simulink model "BodyDynamics"  (R2022b)
settings: Solver=VariableStepAuto  StartTime=0.0  StopTime=60  RelTol=1e-3
values from neighbouring files (symbols this model uses):
  csi_0 = [x_0, z_0, theta_0, u_0, w_0, q_0]'    [Inizializzazione.m]
  dt = double(subs(dt,dt, 0.01))    [Inizializzazione.m]
  is_particle = true    [Inizializzazione.m]
  P_00 = diag([0.1,0.1,0.1,0.1,0.1,0.1])    [Inizializzazione.m]
  Q = diag([var_tau_u, var_tau_w, var_tau_q])    [Inizializzazione.m]
  q_0 = 0    [Inizializzazione.m]
  R = diag([var_y_alpha_m, var_z_m, var_theta_m])    [Inizializzazione.m]
  S = [m , I_y, Damping_matrix(1,1), Damping_matrix(2,2), Damping_matrix(3,3)]    [Inizializzazione.m]
  theta_0 = wrapTo2Pi(rand() * (pi/2) - pi)    [Inizializzazione.m]
  u_0 = 0    [Inizializzazione.m]
  w_0 = 0    [Inizializzazione.m]
  x_0 = rand() * x_boa_1*3/4    [Inizializzazione.m]
  z_0 = rand() * z_boa_2*3/4    [Inizializzazione.m]
  z_boa_2 = 150    [Inizializzazione.m]
libraries: simulink x6
settings Model: Creator=angel  LastModifiedBy=angel
settings DebuggingCC: UnderSpecifiedDimensionMsg=warning
settings ModelReferenceCC: EnableRefExpFcnMdlSchedulingChecks=on

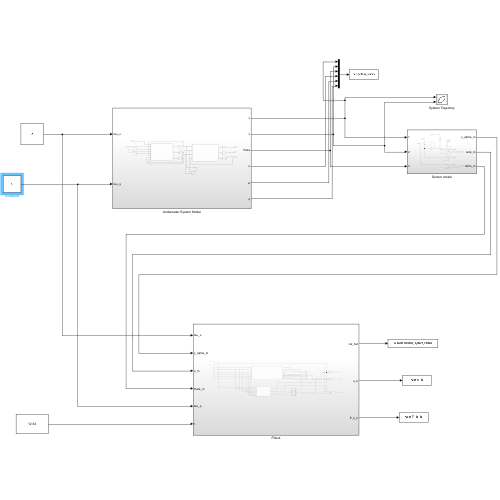
[thumbnail: Simulink's stored preview of the top-level diagram]
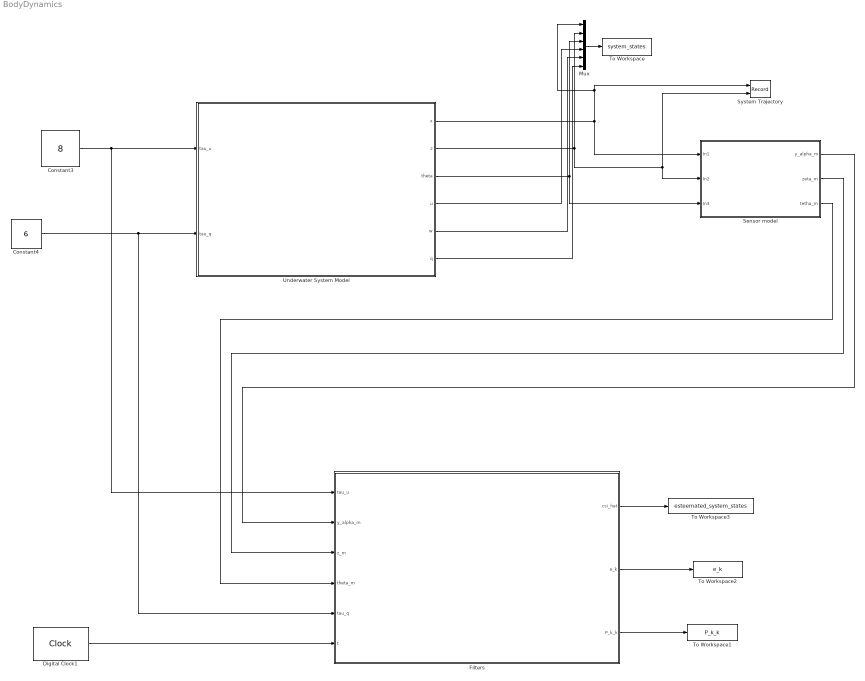
== system BodyDynamics ==
  Constant3 : Constant  Value=8
  Constant4 : Constant  Value=6
  Digital Clock1 : DigitalClock  SampleTime=0.1
  Filters : Subsystem
  Mux : Mux  Inputs=6
  Sensor model : Subsystem
  System Trajectory : Record  FileSettingsInternal="{\"entries\":[{\"content\":{\"excelSettings\":{\"content\":{},\"type\":\"Streamout.ExcelSettings\"}},\"type\":\"Streamout.FileSettingStorage\",\"uuid\":\"5a9cd2f8-3f1b-4377-9d18-0cf4235dc122\"}],\"packageUris\":[\"http://schema.mathworks.com/mf0/streamout_blocks/R2020a\"],\"version\":\"1.0\"}"  Layout=[1 1]  SignalsInternal="{\"entries\":[{\"content\":{\"signals\":[{\"content\":{\"blockPath\":[\"BodyDynamics/System Trajectory\"],\"channel\":[],\"dimensions\":[1],\"domain\":\"BodyDynamics/System Trajectory\",\"lineColor\":\"#ff6929\",\"plots\":[],\"port\":1,\"sid\":[\"\"],\"signalID\":475,\"signalName\":\"Underwater System Model:1\"},\"type\":\"RecordBlkView.Signal\",\"uuid\":\"2e985c3f-a8fe-4c9c-bedf-405b71b3ce1e\"},{\"content\":{\"blockPath\":[\"BodyDynamics/System Trajectory\"],\"channel\":[],\"dimensions\":[1],\"domain\":\"BodyDynamics/System Trajectory\",\"lineColor\":\"#b746ff\",\"plots\":[],\"port\":2,\"sid\":[\"\"],\"signalID\":479,\"signalName\":\"Underwater System Model:2\"},\"type\":\"RecordBlkView.Signal\",\"uuid\":\"8a6af6fa-3ed6-44e8-a576-d0f0524b2a32\"}]},\"type\":\"RecordBlkView.InputSignals\",\"uuid\":\"c673d974-d470-40e6-a6d2-e1dc34d32e7d\"}],\"packageUris\":[\"http://schema.mathworks.com/mf0/streamout_blocks/R2020a\"],\"version\":\"1.0\"}"  VisualizationBindings="{\"xyplotplugin\":{\"info\":[{\"series\":[],\"subplotID\":1}]}}"  CompatibilityTag=XY
  To Workspace : ToWorkspace  VariableName=system_states  SampleTime=dt
  To Workspace1 : ToWorkspace  VariableName=P_k_k  SampleTime=dt
  To Workspace2 : ToWorkspace  VariableName=e_k  SampleTime=dt
  To Workspace3 : ToWorkspace  VariableName=esteemated_system_states  SampleTime=dt
  Underwater System Model : Subsystem
  wires:
  Underwater System Model/1(x) -> System Trajectory/1, Mux/1, Sensor model/1(In1)
  Underwater System Model/2(z) -> System Trajectory/2, Sensor model/2(In2), Mux/2
  Underwater System Model/3(theta) -> Sensor model/3(In3), Mux/3
  Underwater System Model/4(u) -> Mux/4
  Underwater System Model/5(w) -> Mux/5
  Underwater System Model/6(q) -> Mux/6
  Mux/1 -> To Workspace/1
  Constant3/1 -> Filters/1(tau_u), Underwater System Model/1(tau_u)
  Constant4/1 -> Filters/5(tau_q), Underwater System Model/2(tau_q)
  Sensor model/1(y_alpha_m) -> Filters/2(y_alpha_m)
  Sensor model/2(zeta_m) -> Filters/3(z_m)
  Sensor model/3(tetha_m) -> Filters/4(theta_m)
  Digital Clock1/1 -> Filters/6(t)
  Filters/1(csi_hat) -> To Workspace3/1
  Filters/2(e_k) -> To Workspace2/1
  Filters/3(P_k_k) -> To Workspace1/1

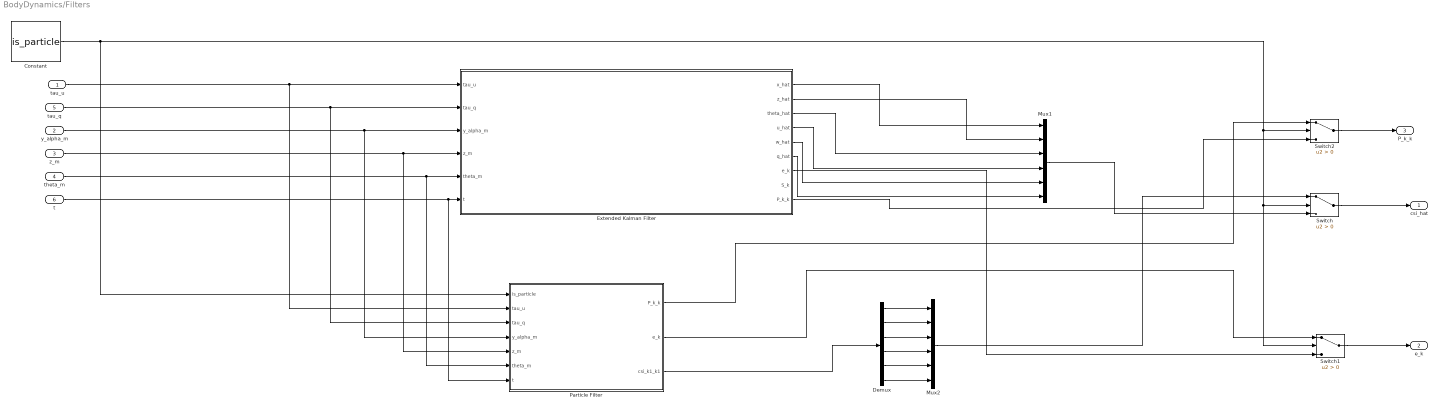
== system BodyDynamics/Filters ==
  tau_u : Inport
  y_alpha_m : Inport  Port=2
  z_m : Inport  Port=3
  theta_m : Inport  Port=4
  tau_q : Inport  Port=5
  t : Inport  Port=6
  Constant : Constant  Value=is_particle
  Demux : Demux  Outputs=6
  Extended Kalman Filter : Subsystem
  Mux1 : Mux  Inputs=6
  Mux2 : Mux  Inputs=6
  Particle Filter : Subsystem
  Switch : Switch  Criteria=u2 > Threshold  SaturateOnIntegerOverflow=off  InputSameDT=off
  Switch1 : Switch  Criteria=u2 > Threshold  SaturateOnIntegerOverflow=off  InputSameDT=off
  Switch2 : Switch  Criteria=u2 > Threshold  SaturateOnIntegerOverflow=off  InputSameDT=off
  csi_hat : Outport
  e_k : Outport  Port=2
  P_k_k : Outport  Port=3
  wires:
  Extended Kalman Filter/4(u_hat) -> Mux1/4
  Extended Kalman Filter/1(x_hat) -> Mux1/1
  Extended Kalman Filter/5(w_hat) -> Mux1/5
  Extended Kalman Filter/2(z_hat) -> Mux1/2
  Demux/4 -> Mux2/4
  Demux/2 -> Mux2/2
  Extended Kalman Filter/6(q_hat) -> Mux1/6
  Demux/6 -> Mux2/6
  Demux/3 -> Mux2/3
  Demux/1 -> Mux2/1
  Extended Kalman Filter/3(theta_hat) -> Mux1/3
  Demux/5 -> Mux2/5
  Mux2/1 -> Switch/1
  Mux1/1 -> Switch/3
  Switch/1 -> csi_hat/1
  Extended Kalman Filter/7(e_k) -> Switch1/3
  Switch1/1 -> e_k/1
  Constant/1 -> Particle Filter/1(is_particle), Switch1/2, Switch/2, Switch2/2
  tau_u/1 -> Particle Filter/2(tau_u), Extended Kalman Filter/1(tau_u)
  tau_q/1 -> Particle Filter/3(tau_q), Extended Kalman Filter/2(tau_q)
  y_alpha_m/1 -> Particle Filter/4(y_alpha_m), Extended Kalman Filter/3(y_alpha_m)
  z_m/1 -> Particle Filter/5(z_m), Extended Kalman Filter/4(z_m)
  theta_m/1 -> Particle Filter/6(theta_m), Extended Kalman Filter/5(theta_m)
  t/1 -> Particle Filter/7(t), Extended Kalman Filter/6(t)
  Extended Kalman Filter/9(P_k_k) -> Switch2/3
  Switch2/1 -> P_k_k/1
  Particle Filter/1(P_k_k) -> Switch2/1
  Particle Filter/2(e_k) -> Switch1/1
  Particle Filter/3(csi_k1_k1) -> Demux/1

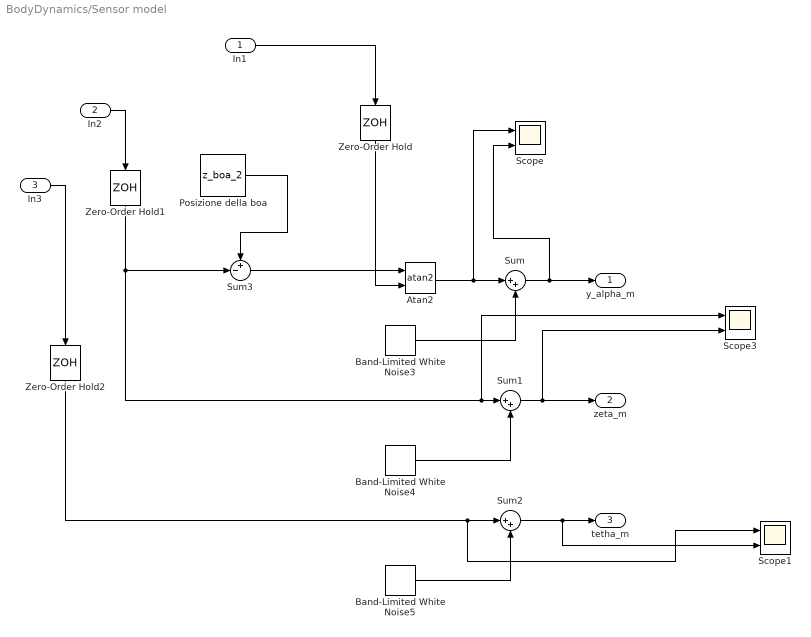
== system BodyDynamics/Sensor model ==
  In1 : Inport
  In2 : Inport  Port=2
  In3 : Inport  Port=3
  Atan2 : Trigonometry  Operator=atan2
  Band-Limited White Noise3 : simulink/Sources/Band-Limited White Noise  Cov=var_y_alpha_m  Ts=dt  seed=[23341]
  Band-Limited White Noise4 : simulink/Sources/Band-Limited White Noise  Cov=var_z_m  Ts=dt  seed=[23341]
  Band-Limited White Noise5 : simulink/Sources/Band-Limited White Noise  Cov=var_theta_m  Ts=dt  seed=[23341]
  Posizione della boa : Constant  Value=z_boa_2
  Scope : Scope  NumInputPorts=2
  Scope1 : Scope  NumInputPorts=2
  Scope3 : Scope  NumInputPorts=2
  Sum : Sum  Inputs=|++
  Sum1 : Sum  Inputs=|++
  Sum2 : Sum  Inputs=|++
  Sum3 : Sum  Inputs=+-|
  Zero-Order Hold : ZeroOrderHold  SampleTime=dt
  Zero-Order Hold1 : ZeroOrderHold  SampleTime=dt
  Zero-Order Hold2 : ZeroOrderHold  SampleTime=dt
  y_alpha_m : Outport
  zeta_m : Outport  Port=2
  tetha_m : Outport  Port=3
  wires:
  In3/1 -> Zero-Order Hold2/1
  In1/1 -> Zero-Order Hold/1
  Sum2/1 -> Scope1/2, tetha_m/1
  Sum1/1 -> Scope3/2, zeta_m/1
  In2/1 -> Zero-Order Hold1/1
  Band-Limited White Noise3/1 -> Sum/2
  Band-Limited White Noise4/1 -> Sum1/2
  Band-Limited White Noise5/1 -> Sum2/2
  Zero-Order Hold/1 -> Atan2/2
  Zero-Order Hold1/1 -> Sum3/2, Scope3/1, Sum1/1
  Zero-Order Hold2/1 -> Scope1/1, Sum2/1
  Posizione della boa/1 -> Sum3/1
  Sum3/1 -> Atan2/1
  Atan2/1 -> Scope/1, Sum/1
  Sum/1 -> y_alpha_m/1, Scope/2

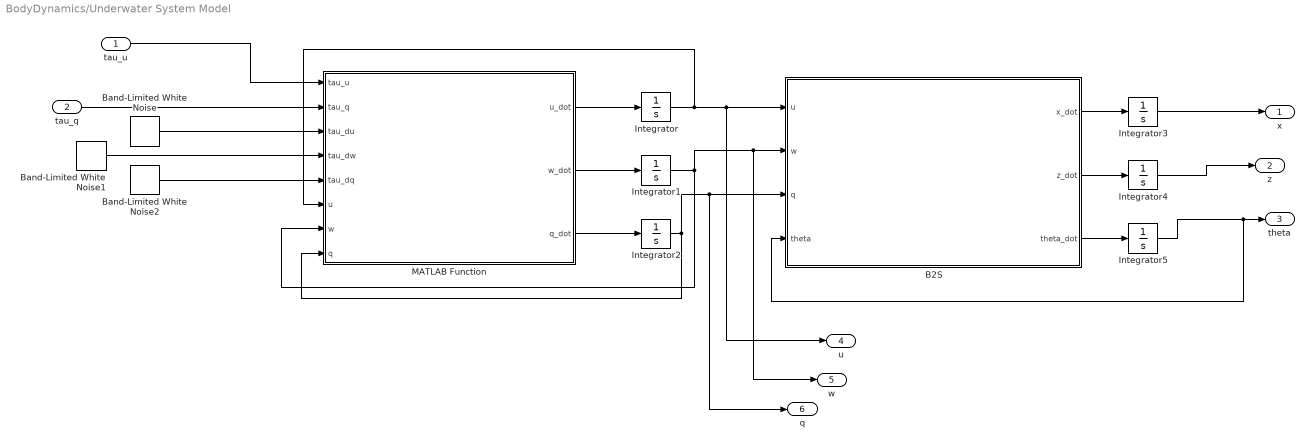
== system BodyDynamics/Underwater System Model ==
  tau_u : Inport
  tau_q : Inport  Port=2
  B2S : MATLAB Function  TreatAsAtomicUnit=on
  Band-Limited White Noise : simulink/Sources/Band-Limited White Noise  Cov=var_tau_u  Ts=dt  seed=[23341]
  Band-Limited White Noise1 : simulink/Sources/Band-Limited White Noise  Cov=var_tau_w  Ts=dt  seed=[23341]
  Band-Limited White Noise2 : simulink/Sources/Band-Limited White Noise  Cov=var_tau_q  Ts=dt  seed=[23341]
  Integrator : Integrator  InitialCondition=u_0
  Integrator1 : Integrator  InitialCondition=w_0
  Integrator2 : Integrator  InitialCondition=q_0
  Integrator3 : Integrator  InitialCondition=x_0
  Integrator4 : Integrator  InitialCondition=z_0
  Integrator5 : Integrator  InitialCondition=theta_0  WrappedStateUpperValue=2*pi  WrappedStateLowerValue=0
  MATLAB Function : MATLAB Function  TreatAsAtomicUnit=on  mask{S=S}
      mask prompts: S "Costanti del sistema"
  x : Outport
  z : Outport  Port=2
  theta : Outport  Port=3
  u : Outport  Port=4
  w : Outport  Port=5
  q : Outport  Port=6
  wires:
  B2S/2(z_dot) -> Integrator4/1
  Integrator1/1 -> MATLAB Function/7(w), w/1, B2S/2(w)
  Band-Limited White Noise2/1 -> MATLAB Function/5(tau_dq)
  B2S/3(theta_dot) -> Integrator5/1
  MATLAB Function/2(w_dot) -> Integrator1/1
  Integrator/1 -> MATLAB Function/6(u), B2S/1(u), u/1
  B2S/1(x_dot) -> Integrator3/1
  MATLAB Function/3(q_dot) -> Integrator2/1
  MATLAB Function/1(u_dot) -> Integrator/1
  Band-Limited White Noise1/1 -> MATLAB Function/4(tau_dw)
  tau_u/1 -> MATLAB Function/1(tau_u)
  Integrator2/1 -> MATLAB Function/8(q), q/1, B2S/3(q)
  Band-Limited White Noise/1 -> MATLAB Function/3(tau_du)
  Integrator5/1 -> B2S/4(theta), theta/1
  Integrator3/1 -> x/1
  Integrator4/1 -> z/1
  tau_q/1 -> MATLAB Function/2(tau_q)

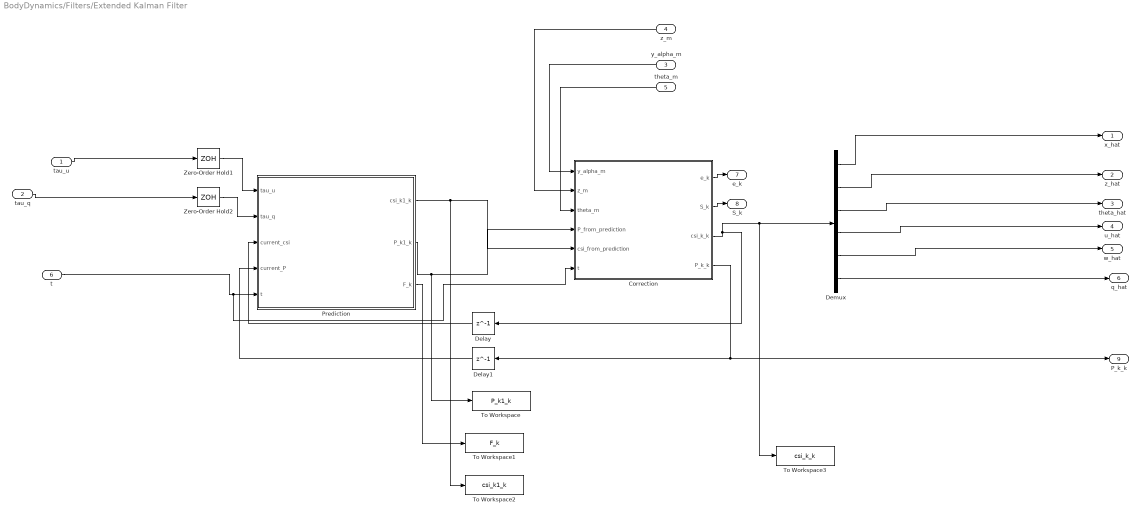
== system BodyDynamics/Filters/Extended Kalman Filter ==
  tau_u : Inport
  tau_q : Inport  Port=2
  y_alpha_m : Inport  Port=3
  z_m : Inport  Port=4
  theta_m : Inport  Port=5
  t : Inport  Port=6
  Correction : MATLAB Function  TreatAsAtomicUnit=on  mask{R=R, z_boa_2=z_boa_2}
      mask prompts: R "Matrice varianze dei distrubi"; z_boa_2 "Profondità della boa 2"
  Delay : Delay  DelayLength=1  InitialCondition=0  SampleTime=dt
  Delay1 : Delay  DelayLength=1  InitialCondition=0  SampleTime=dt
  Demux : Demux  Outputs=6
  Prediction : MATLAB Function  TreatAsAtomicUnit=on  mask{csi_0=csi_0, Q=Q, P_00=P_00, dt=dt, S=S}
      mask prompts: csi_0 "stima iniziale di csi"; Q "Matrice delle varianze dei disturbi di ingresso"; P_00 "Valore iniziale di P"; dt "Sampling time"; S "Parametri del sistema"
  To Workspace : ToWorkspace  VariableName=P_k1_k  SampleTime=dt
  To Workspace1 : ToWorkspace  VariableName=F_k  SampleTime=dt
  To Workspace2 : ToWorkspace  VariableName=csi_k1_k  SampleTime=dt
  To Workspace3 : ToWorkspace  VariableName=csi_k_k  SampleTime=dt
  Zero-Order Hold1 : ZeroOrderHold  SampleTime=dt
  Zero-Order Hold2 : ZeroOrderHold  SampleTime=dt
  x_hat : Outport
  z_hat : Outport  Port=2
  theta_hat : Outport  Port=3
  u_hat : Outport  Port=4
  w_hat : Outport  Port=5
  q_hat : Outport  Port=6
  e_k : Outport  Port=7
  S_k : Outport  Port=8
  P_k_k : Outport  Port=9
  wires:
  Correction/3(csi_k_k) -> Delay/1, To Workspace3/1, Demux/1
  Demux/6 -> q_hat/1
  Correction/4(P_k_k) -> P_k_k/1, Delay1/1
  Demux/3 -> theta_hat/1
  Delay/1 -> Prediction/3(current_csi)
  Delay1/1 -> Prediction/4(current_P)
  Prediction/1(csi_k1_k) -> Correction/5(csi_from_prediction), To Workspace2/1
  tau_q/1 -> Zero-Order Hold2/1
  theta_m/1 -> Correction/3(theta_m)
  Demux/4 -> u_hat/1
  z_m/1 -> Correction/2(z_m)
  Correction/2(S_k) -> S_k/1
  Zero-Order Hold2/1 -> Prediction/2(tau_q)
  Prediction/2(P_k1_k) -> To Workspace/1, Correction/4(P_from_prediction)
  Zero-Order Hold1/1 -> Prediction/1(tau_u)
  y_alpha_m/1 -> Correction/1(y_alpha_m)
  tau_u/1 -> Zero-Order Hold1/1
  t/1 -> Correction/6(t), Prediction/5(t)
  Demux/1 -> x_hat/1
  Demux/2 -> z_hat/1
  Demux/5 -> w_hat/1
  Correction/1(e_k) -> e_k/1
  Prediction/3(F_k) -> To Workspace1/1

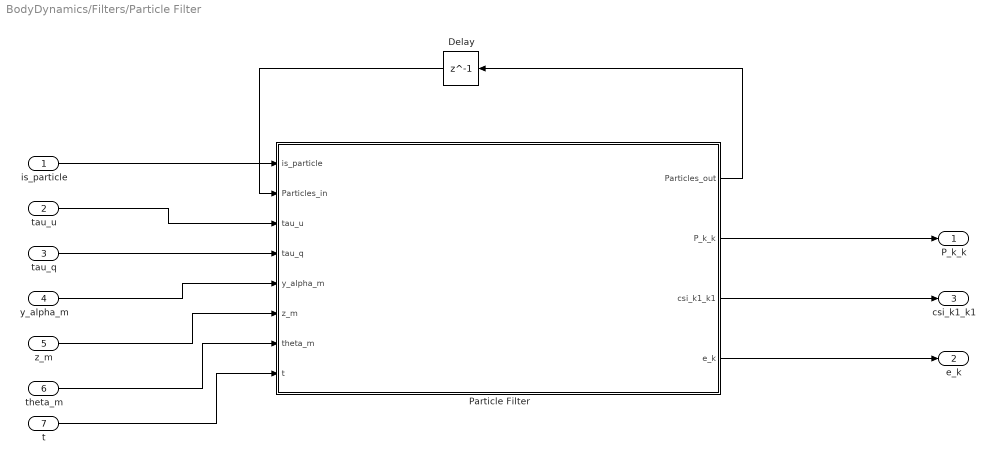
== system BodyDynamics/Filters/Particle Filter ==
  is_particle : Inport
  tau_u : Inport  Port=2
  tau_q : Inport  Port=3
  y_alpha_m : Inport  Port=4
  z_m : Inport  Port=5
  theta_m : Inport  Port=6
  t : Inport  Port=7
  Delay : Delay  DelayLength=1  InitialCondition=0  SampleTime=dt
  Particle Filter : MATLAB Function  TreatAsAtomicUnit=on  mask{S=S, Q=Q, R=R, dt=dt, csi_0=csi_0, z_boa_2=z_boa_2}
      mask prompts: S "Costanti del sistema"; Q "Matrice delle varianze dei disturbi in ingresso"; R "Matrice delle varianze dei disturbi in uscita"; dt "Tempo di campionamento"; csi_0 "Stato iniziale"; z_boa_2 "Profondità boa"
  P_k_k : Outport
  e_k : Outport  Port=2
  csi_k1_k1 : Outport  Port=3
  wires:
  Particle Filter/3(csi_k1_k1) -> csi_k1_k1/1
  Delay/1 -> Particle Filter/2(Particles_in)
  Particle Filter/1(Particles_out) -> Delay/1
  Particle Filter/4(e_k) -> e_k/1
  z_m/1 -> Particle Filter/6(z_m)
  t/1 -> Particle Filter/8(t)
  theta_m/1 -> Particle Filter/7(theta_m)
  tau_u/1 -> Particle Filter/3(tau_u)
  tau_q/1 -> Particle Filter/4(tau_q)
  Particle Filter/2(P_k_k) -> P_k_k/1
  is_particle/1 -> Particle Filter/1(is_particle)
  y_alpha_m/1 -> Particle Filter/5(y_alpha_m)

== matlab function BodyDynamics/Filters/Particle Filter/Particle Filter ==
  data: is_particle input; Particles_out output; P_k_k output; Particles_in input size=[6,20000]; tau_u input; tau_q input; y_alpha_m input; z_m input; theta_m input; t input; csi_k1_k1 output; z_boa_2 parameter; R parameter; Q parameter; S parameter; csi_0 parameter; dt parameter; e_k output size=[3,1]
function [Particles_out, P_k_k, csi_k1_k1, e_k] = Particle_Filter(is_particle, Particles_in, tau_u, tau_q, y_alpha_m, z_m, theta_m, t,z_boa_2, R, Q, S, csi_0, dt)
      
    m = S(1);
    I_y = S(2);
    Damping_matrix = diag([S(3),S(4),S(5)]);
    
    N = 20000;              % Numero di particelle che generiamo 
    
    if(is_particle)
        if(t == 0)               % Generazione particelle nell'istante t=0
    
            % Definiamo i range di incertezza
            
            range_x = 3;
            range_z = 3;
            range_theta = 0.01;
            range_u = 0.01;
            range_w = 0.01;
            range_q = 0.01;
    
            % Generiamo le particelle per ogni variabile del problema
    
            particles_x = rand(1,N)*range_x + (csi_0(1)-range_x/2);
            particles_z = rand(1,N)*range_z + (csi_0(2)-range_z/2);
            particles_theta = rand(1,N)*range_theta + (csi_0(3)-range_theta/2);
            particles_u = rand(1,N)*range_u + (csi_0(4)-range_u/2);
            particles_w = rand(1,N)*range_w + (csi_0(5)-range_w/2);
            particles_q = rand(1,N)*range_q + (csi_0(6)-range_q/2);
            Particles_k1_k = [particles_x; particles_z; particles_theta; particles_u; particles_w; particles_q];
            w_posteriori = ones(1,N)/N;
        
        else
        
            % Definizione del vettori vuoti da usare nell'algoritmo
            Particles_k1_k = zeros(size(Particles_in));
            e = zeros(3,N);
            w_posteriori = zeros(1,N);
            e_y_alpha_m = zeros(1,N);
            e_z_m = zeros(1,N);
            e_theta_m = zeros(1,N);
            Particles_k_k = Particles_in;
            for i=1:N               % Per ogni i-esima particella viene fatta predizione e correzione
                x = Particles_k_k(1,i);
                z = Particles_k_k(2,i);
                theta = wrapToPi(Particles_k_k(3,i));
                u = Particles_k_k(4,i);
                w = Particles_k_k(5,i);
                q = Particles_k_k(6,i);
                tau_du = randn()*Q(1,1);
                tau_dw = randn()*Q(2,2);
                tau_dq = randn()*Q(3,3);
        
                csi_dot = [ cos(conj(theta))*conj(u) + sin(conj(theta))*conj(w)
                    cos(conj(theta))*conj(w) - sin(conj(theta))*conj(u)
                    conj(q)
                    (conj(tau_u) + conj(tau_du) - conj(Damping_matrix(1,1))*conj(u) - conj(m)*conj(q)*conj(w))/conj(m)
                    (conj(tau_dw) - conj(Damping_matrix(2,2))*conj(w) + conj(m)*conj(q)*conj(u))/conj(m)
                    (conj(tau_q) + conj(tau_dq) - conj(Damping_matrix(3,3))*conj(q))/conj(I_y)];
                
                % Predizione
                Particles_k1_k(:,i) = Particles_k_k(:,i) + dt*csi_dot;
                
                e_y_alpha_m(i) = y_alpha_m - atan2(z_boa_2 - Particles_k1_k(2,i), Particles_k1_k(1,i));
                e_z_m(i) = z_m - Particles_k1_k(2,i);
                e_theta_m(i) = theta_m - Particles_k1_k(3,i);
                e(:,i) = [e_y_alpha_m(i) e_z_m(i) e_theta_m(i)]';
        
                % Correzione
                w_posteriori(i) = double(exp(-1/2*(e(:,i)'*inv(R)*e(:,i))));     % Pesi a posteriori
            end
            % Nel caso in cui la verosomiglianza sia nulla
            % (per troncamentro) poniamo i pesi come di pdf uniforme
            if(sum(w_posteriori) == 0)
                w_posteriori = ones(1,N)/N;
             end
        end
        w_posteriori_norm = w_posteriori./sum(w_posteriori);        % Normalizzazione dei pesi
        csi_k1_k1 = zeros(6,1);

        % Calcolo della stima (EAP/MMSE)
        for k=1:N
            csi_k1_k1 = csi_k1_k1 + w_posteriori_norm(k).*Particles_k1_k(:,k);
        end

        % Calcolo dell'innovazione
        e_y_alpha = y_alpha_m - atan2(z_boa_2 - csi_k1_k1(2), csi_k1_k1(1));
        e_z = z_m - csi_k1_k1(2);
        e_theta = theta_m - csi_k1_k1(3);
    
        % Resampling (Algoritmo della roulette)
        Resample = zeros(size(Particles_in));                
        c = zeros(1,N);
        u = zeros(1,N);
        c(1) = w_posteriori_norm(1);
        for i=2:N
            c(i) = c(i-1) + w_posteriori_norm(i);
        end
        u(1) = rand()/N;
        i = 1;
        for j=1:N
            while(u(j)>c(i))
                i=i+1;
            end
            Resample(:,j) = Particles_k1_k(:,i);
            if(j<N)
                u(j+1) = u(j) + 1/N;
            end
        end
        
        % Calcolo della varianza di stima
        P_k_k = zeros(6,6);

        for i=1:N
            
           P_k_k = P_k_k + w_posteriori_norm(i).*(Particles_k1_k(:,i) - csi_k1_k1)*(Particles_k1_k(:,i) - csi_k1_k1)';

        end
        
        % Particelle in uscita (sporcate con rumore bianco)
        Particles_out = diag([0.01 0.01 0.001 0 0 0])*randn(6,N) + Resample;
        
        e_k = [e_y_alpha, e_z, e_theta]';
    else
        % Nel caso in cui non usiamo il Particle Filter andiamo a dare in
        % uscita segnali nulli
        Particles_out = zeros(6,N);
        csi_k1_k1 = zeros(6,1);
        e_k = zeros(3,1);
        P_k_k = zeros(6,6);

    end
end

== matlab function BodyDynamics/Underwater System Model/B2S ==
  data: u input; x_dot output; w input; q input; theta input; z_dot output; theta_dot output
function [x_dot, z_dot, theta_dot] = BodyToSpatial(u, w, q, theta)
    theta = wrapToPi(theta);
    R = [cos(theta) sin(theta) 0; -sin(theta) cos(theta) 0; 0 0 1];   % matrice di rotazione B2S
    S_spatial = R*[u w q]';
    x_dot = S_spatial(1);
    z_dot = S_spatial(2);
    theta_dot = S_spatial(3);
end

== matlab function BodyDynamics/Underwater System Model/MATLAB Function ==
  data: tau_u input; tau_q input; tau_du input; tau_dw input; tau_dq input; u input; u_dot output size=1; w input; q input; w_dot output size=1; q_dot output size=1; S parameter
function [u_dot, w_dot, q_dot] = BodyDynamics(tau_u, tau_q, tau_du, tau_dw, tau_dq, u, w, q, S)
    
    % Parametri del sistema
    
    m = S(1);
    I_y = S(2);
    Damping_matrix = diag([S(3),S(4),S(5)]);
    
    B=[m 0 0; 0 m 0; 0 0 I_y];          % Matrice di massa
    C=[Damping_matrix(1,1) 0 m*w;
       0 Damping_matrix(2,2) -m*u ;
       -m*w m*u Damping_matrix(3,3)];   % Matrice dei termini di Coriolis
    Tau=[tau_u;0; tau_q];
    Tau_d=[tau_du; tau_dw; tau_dq];
    S_Body=[u;w;q];
    S_Body_dot = inv(B)*(Tau+Tau_d-C*S_Body);
    u_dot= S_Body_dot(1);
    w_dot=S_Body_dot(2);
    q_dot=S_Body_dot(3);


end

== matlab function BodyDynamics/Filters/Extended Kalman Filter/Prediction ==
  data: tau_u input; tau_q input; csi_k1_k output; csi_0 parameter; current_csi input; current_P input; t input; P_k1_k output; P_00 parameter; Q parameter; dt parameter; S parameter; F_k output
function [csi_k1_k, P_k1_k, F_k] = Prediction(tau_u, tau_q, csi_0, current_csi, current_P, t, P_00, Q, dt, S)
    
    % Parametri del sistema

    m = S(1);
    I_y = S(2);
    Damping_matrix = diag([S(3),S(4),S(5)]);

    % Inserimento del valore iniziale in t = 0

    if t == 0                          
        csi_k_k = csi_0 + P_00*randn(6,1);
        P_k_k = P_00;
    else 
        csi_k_k = current_csi;        % current_csi è il valore della stima corretta al passo corrente
        P_k_k = current_P;
    end
    
    % Valori delle variabili di stima dello stato da usare nel calcolo dei Jacobiani

    x = csi_k_k(1);
    z = csi_k_k(2);
    theta = wrapToPi(csi_k_k(3));
    u = csi_k_k(4);
    w = csi_k_k(5);
    q = csi_k_k(6);
    tau_du = 0;
    tau_dw = 0;
    tau_dq = 0;

    % Calcolo del Jacobiano del modello dinamico rispetto alle stime 

    F_k = [1 0 dt*(cos(conj(theta))*conj(w)-sin(conj(theta))*conj(u)) dt*cos(conj(theta)) dt*sin(conj(theta)) 0
           0 1 -dt*(cos(conj(theta))*conj(u)+sin(conj(theta))*conj(w)) -dt*sin(conj(theta)) dt*cos(conj(theta)) 0
           0 0 1 0 0 dt
           0 0 0 1-(dt*conj(Damping_matrix(1,1)))/conj(m) -dt*conj(q) -dt*conj(w)
           0 0 0  dt*conj(q) 1-(dt*conj(Damping_matrix(2,2)))/conj(m)  dt*conj(u)
           0 0 0 0 0 1-(dt*conj(Damping_matrix(3,3)))/conj(I_y)];


    % Jacobiano del modello dinamico rispetto ai disturbi in ingresso

    D_k = [   0,    0,       0
              0,    0,       0
              0,    0,       0
          dt/m,    0,       0
              0, dt/m,       0
              0,    0, dt/I_y];

    % Calcolo della derivata temporale delle variabili di stato

    csi_dot = [ cos(conj(theta))*conj(u) + sin(conj(theta))*conj(w)
                cos(conj(theta))*conj(w) - sin(conj(theta))*conj(u)
                conj(q)
                (conj(tau_u) + conj(tau_du) - conj(Damping_matrix(1,1))*conj(u) - conj(m)*conj(q)*conj(w))/conj(m)
                (conj(tau_dw) - conj(Damping_matrix(2,2))*conj(w) + conj(m)*conj(q)*conj(u))/conj(m)
                (conj(tau_q) + conj(tau_dq) - conj(Damping_matrix(3,3))*conj(q))/conj(I_y)];
    
    % Stima predetta
    if t == 0
        csi_k1_k = csi_k_k;
        csi_k1_k(3) = (csi_k1_k(3));
        P_k1_k = P_00;
    else
        csi_k1_k = csi_k_k + dt * csi_dot;
        csi_k1_k(3) = (csi_k1_k(3));
        P_k1_k=(F_k*P_k_k*(F_k)')+(D_k*Q*(D_k)');
    end
end

== matlab function BodyDynamics/Filters/Extended Kalman Filter/Correction ==
  data: y_alpha_m input; e_k output size=[3,1]; z_m input; theta_m input; P_from_prediction input; csi_from_prediction input; S_k output size=[3,3]; csi_k_k output size=[6,1]; P_k_k output size=[6,6]; R parameter; z_boa_2 parameter; t input
function [e_k, S_k, csi_k_k, P_k_k] = Correction(y_alpha_m, z_m, theta_m, P_from_prediction, csi_from_prediction, R, z_boa_2,t)
    
    % Vettore delle misure in uscita dal sensore

    y_alpha_m = (y_alpha_m);
    theta_m = (theta_m);
    y_k=[y_alpha_m, z_m, theta_m]';
    
    % Stima predetta

    csi_k_kmeno1 = csi_from_prediction;
    P_k_kmeno1 = P_from_prediction; 
    
    x = csi_k_kmeno1(1);
    z = csi_k_kmeno1(2);
    theta = csi_k_kmeno1(3);    
    u = csi_k_kmeno1(4);
    w = csi_k_kmeno1(5);
    q = csi_k_kmeno1(6);
    v_y_alpha_m = 0;
    v_z_m = 0;
    v_theta_m = 0;
    
    % calcoliamo le matrici in Matlab e riportiamo qui i risultati

    % Innovazione

    e_k = y_k - [(atan2(z_boa_2 - z, x))+(v_y_alpha_m); (v_z_m)+(z); (theta)+(v_theta_m)];
    
    % Jacobiano del modello di misura rispetto alle stime a priori

    H_k = [-(imag(x) - real(z) + z_boa_2)/((imag(z) + real(x))^2 + (imag(x) - real(z) + z_boa_2)^2), -(imag(z) + real(x))/((imag(z) + real(x))^2 + (imag(x) - real(z) + 150)^2), 0, 0, 0, 0
           0, 1, 0, 0, 0, 0
           0, 0, 1, 0, 0, 0];

    % Jacobiano del modello di misura rispetto all rumore di misura

    M_k = eye(3);

    % Covarianza dell'innovazione

    S_k=H_k*P_k_kmeno1*(H_k)'+M_k*R*(M_k)';

    % Guadagno di correzione

    L_k=(P_k_kmeno1*(H_k)')/(S_k);
    
    if(t==0)
        csi_k_k = csi_k_kmeno1;
        P_k_k = P_k_kmeno1;
    
    else    
        % Stima corretta (a posteriori)
    
        csi_k_k = csi_k_kmeno1+L_k*e_k;
    
        % Varianza dell'errore di stima a posteriori
        %%% Si può usare la forma di Joseph? %%%
        P_k_k=P_k_kmeno1-(L_k*S_k*(L_k)');
    end
    
end
